simulink model "main"  (R2024b)
settings: Solver=VariableStepAuto  StartTime=0.0  StopTime=10.0  RelTol=1e-3
undefined symbols (not defined in the file): b1, b2, k, m1, m2
settings Model: Creator=bardi  LastModifiedBy=bardi
settings DataIOCC: LoggingToFile=on

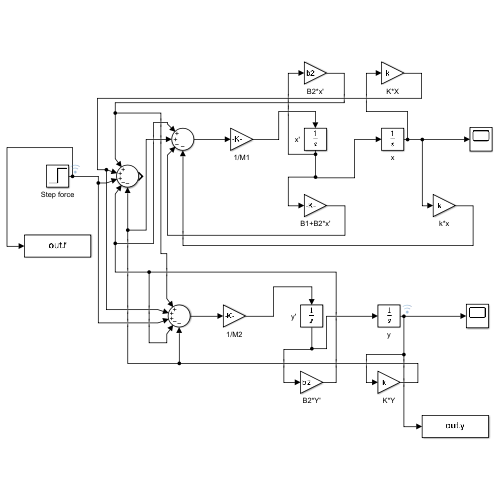
[thumbnail: Simulink's stored preview of the top-level diagram]
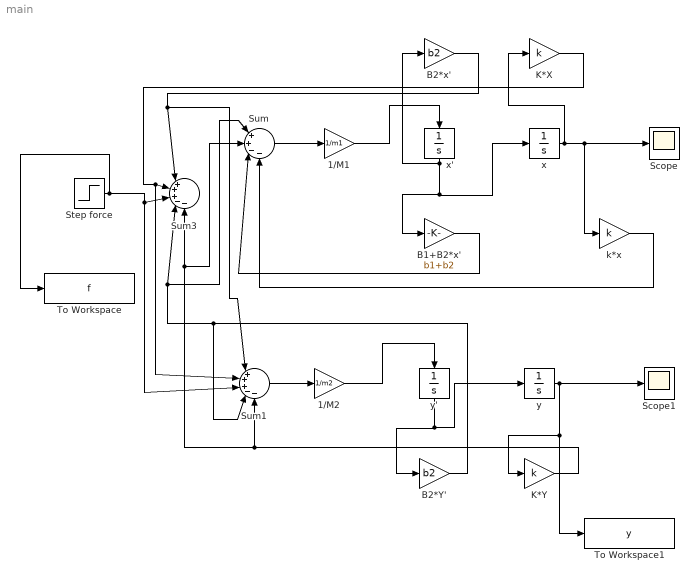
== system main ==
  1/M1 : Gain  Gain=1/m1
  1/M2 : Gain  Gain=1/m2
  B1+B2*x' : Gain  Gain=b1+b2
  B2*Y' : Gain  Gain=b2
  B2*x' : Gain  Gain=b2
  K*X : Gain  Gain=k
  K*Y : Gain  Gain=k
  Scope : Scope
  Scope1 : Scope
  Step force : Step  After=10  SampleTime=0
  Sum : Sum  Inputs=|++--
  Sum1 : Sum  Inputs=|+++--
  Sum3 : Sum  Inputs=|+++--
  To Workspace : ToWorkspace  VariableName=f  SaveFormat=Structure With Time  SampleTime=-1
  To Workspace1 : ToWorkspace  VariableName=y  SaveFormat=Structure With Time  SampleTime=-1
  k*x : Gain  Gain=k
  x : Integrator
  x' : Integrator
  y : Integrator
  y' : Integrator
  wires:
  x'/1 -> B2*x'/1, x/1, B1+B2*x'/1
  Sum/1 -> 1/M1/1
  1/M1/1 -> x'/1
  y'/1 -> y/1, B2*Y'/1
  1/M2/1 -> y'/1
  Sum1/1 -> 1/M2/1
  x/1 -> K*X/1, k*x/1, Scope/1
  y/1 -> To Workspace1/1, K*Y/1, Scope1/1
  k*x/1 -> Sum/4
  B1+B2*x'/1 -> Sum/3
  B2*x'/1 -> Sum3/1, Sum1/1
  K*X/1 -> Sum1/2, Sum3/2
  Step force/1 -> To Workspace/1, Sum3/3, Sum1/3
  B2*Y'/1 -> Sum1/4, Sum3/4, Sum/1
  K*Y/1 -> Sum1/5, Sum3/5, Sum/2
